simulink model "Ejercicio2_09_03_17"  (R2013a)
settings: Solver=ode45  StartTime=0.0  StopTime=10.0  RelTol=1e-3
libraries: powerlib x11, powerlib_meascontrol x4
settings Model: Creator=Miguel  LastModifiedBy=Miguel

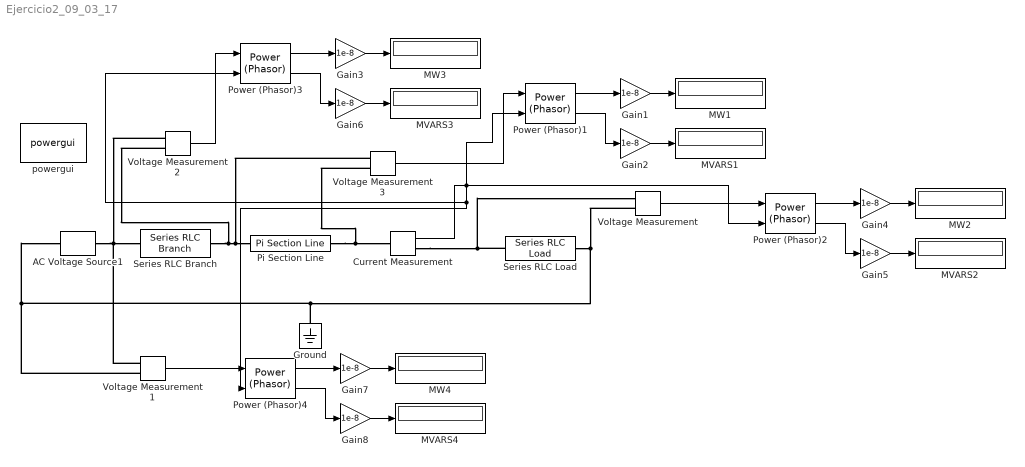
== system Ejercicio2_09_03_17 ==
  AC Voltage Source1 : powerlib/Electrical Sources/AC Voltage Source  Amplitude=114588.6594*sqrt(2)  Phase=1.795612043  Frequency=60  SampleTime=0  Measurements=Voltage
  Current Measurement : powerlib/Measurements/Current Measurement  PhasorSimulation=on  OutputType=Complex  PSBequivalent=0
  Gain{1..8} (8 alike) : Gain  Gain=1e-8
  Ground : powerlib/Elements/Ground  LConnTagsString=a
  MVARS{1..4} (4 alike) : Display
  MW{1..4} (4 alike) : Display
  Pi Section Line : powerlib/Elements/Pi Section Line  LConnTagsString=__new0  RConnTagsString=__new0  Frequency=60  Resistance=0.2  Inductance=0.43/(2*pi*60)  Capacitance=2.6e-6/(2*pi*60)  Length=60  PiSections=1  Measurements=None
      settings: AttributesFormatString=\n
  Power (Phasor){1..4} (4 alike) : powerlib_meascontrol/Measurements/Power (Phasor)
  Series RLC Branch : powerlib/Elements/Series RLC Branch  LConnTagsString=__new0  RConnTagsString=__new0  BranchType=L  Resistance=1  Inductance=1e-9  SetiL0=off  InitialCurrent=0  Capacitance=1e-6  Setx0=off  InitialVoltage=0  Measurements=None
  Series RLC Load : powerlib/Elements/Series RLC Load  LConnTagsString=a  RConnTagsString=__new0  NominalVoltage=110e3  NominalFrequency=60  ActivePower=20e6  InductivePower=10e6  CapacitivePower=0  Setx0=off  InitialVoltage=0  SetiL0=off  InitialCurrent=0  Measurements=None
  Voltage Measurement{,1..3} (4 alike) : powerlib/Measurements/Voltage Measurement  PhasorSimulation=on  OutputType=Complex  PSBequivalent=0
  powergui : powerlib/powergui  Priority=1  SimulationMode=Phasor  SolverType=Tustin  SampleTime=50e-6  frequency=60  SPID=off  DisableSnubberDevices=off  DisableRonSwitches=off  DisableVfSwitches=off  SwTol=0  Interpol=off  DisplayEquations=off  frequencyindice=60  Pbase=100e6  ErrMax=1e-4  Iterations=50  UnitsV=kV  UnitsW=MW  FunctionMessages=off  echomessages=off  HookPort=off  EnableUseOfTLC=off  x0status=blocks  RestoreLinks=warning  ResistiveCurrentMeasurement=off  Frange=[0:2:500]  Ylog=off  Xlog=on  ShowGrid=off  save=off  variable=ZData  ZoomFFT=off  StartTime=0.0  cycles=1  DisplayStyle=1  fundamental=60  FreqAxis=off  MaxFrequency=1000  frequencyindicesteady=1  RmsSteady=2  display=off  Ts=0  methode=off
  wires:
  Power (Phasor)2/1 -> Gain4/1
  Power (Phasor)2/2 -> Gain5/1
  Gain4/1 -> MW2/1
  Gain5/1 -> MVARS2/1
  Voltage Measurement/1 -> Power (Phasor)2/1
  Current Measurement/1 -> Power (Phasor)1/2, Power (Phasor)4/2, Power (Phasor)3/2, Power (Phasor)2/2
  Power (Phasor)1/1 -> Gain1/1
  Power (Phasor)1/2 -> Gain2/1
  Gain1/1 -> MW1/1
  Gain2/1 -> MVARS1/1
  Power (Phasor)3/1 -> Gain3/1
  Power (Phasor)3/2 -> Gain6/1
  Gain3/1 -> MW3/1
  Gain6/1 -> MVARS3/1
  Voltage Measurement2/1 -> Power (Phasor)3/1
  Voltage Measurement3/1 -> Power (Phasor)1/1
  Power (Phasor)4/1 -> Gain7/1
  Power (Phasor)4/2 -> Gain8/1
  Gain7/1 -> MW4/1
  Gain8/1 -> MVARS4/1
  Voltage Measurement1/1 -> Power (Phasor)4/1
  connections:
  Series RLC Load/RConn1 -- Voltage Measurement/LConn2 -- Ground/LConn1 -- AC Voltage Source1/LConn1 -- Voltage Measurement1/LConn2
  Series RLC Load/LConn1 -- Current Measurement/RConn1 -- Voltage Measurement/LConn1
  Pi Section Line/RConn1 -- Voltage Measurement3/LConn2 -- Current Measurement/LConn1
  Series RLC Branch/RConn1 -- Voltage Measurement2/LConn2 -- Voltage Measurement3/LConn1 -- Pi Section Line/LConn1
  AC Voltage Source1/RConn1 -- Voltage Measurement2/LConn1 -- Voltage Measurement1/LConn1 -- Series RLC Branch/LConn1
